simulink model "M182_Lab5"  (R2019b)
settings: Solver=VariableStepAuto  StartTime=0.0  StopTime=10000  RelTol=1e-3
libraries: simulink x1
settings Model: Creator=scjcb  LastModifiedBy=scjcb

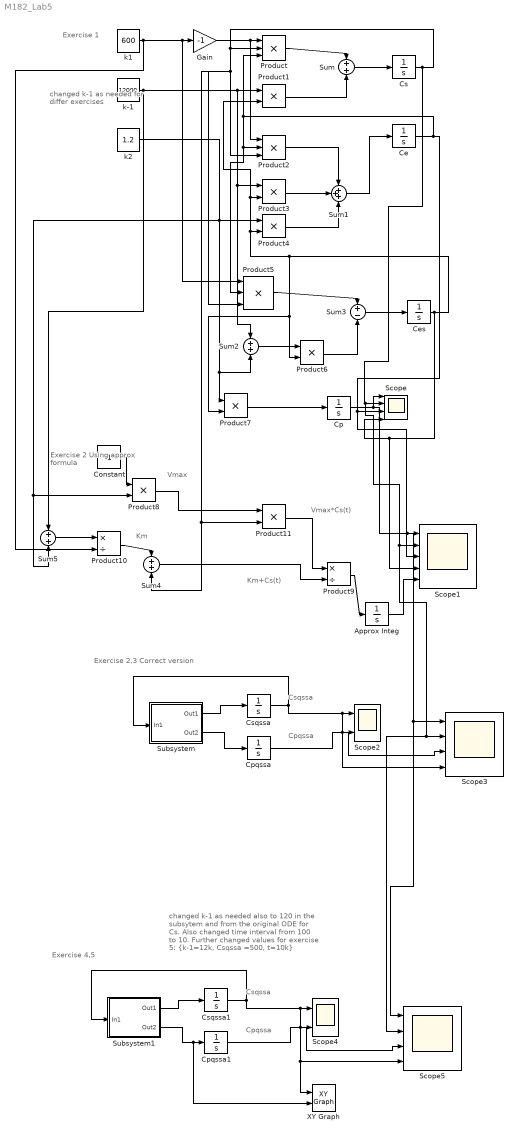
== system M182_Lab5 ==
  note: changed k-1 as needed also
      | to 120 in the subsytem and from
      | the original ODE for Cs. Also changed
      | time interval from 100 to 10.
      | Further changed values for exercise 5:
      | {k-1=12k, Csqssa =500, t=10k}
  note: changed k-1 as
      | needed for
      | differ exercises
  note: Exercise 2,3 Correct version
  note: Cpqssa
  note: Csqssa
  note: Vmax*Cs(t)
  note: Km+Cs(t)
  note: Vmax
  note: Km
  note: Exercise 2
      | Using
      | approx formula
  note: Exercise 1
  note: Cpqssa
  note: Exercise 4,5
  note: Csqssa
  Approx Integ : Integrator
  Ce : Integrator  InitialCondition=1
  Ces : Integrator
  Constant : Constant
  Cp : Integrator
  Cpqssa : Integrator
  Cpqssa1 : Integrator
  Cs : Integrator  InitialCondition=1
  Csqssa : Integrator  InitialCondition=1
  Csqssa1 : Integrator  InitialCondition=500
  Gain : Gain  Gain=-1
  Product : Product  Inputs=3
  Product1 : Product
  Product10 : Product  Inputs=*/
  Product{3..4,6..8,11} (6 alike) : Product  Inputs=**
  Product2 : Product  Inputs=***
  Product5 : Product  Inputs=***
  Product9 : Product  Inputs=*/
  Scope : Scope  NumInputPorts=4
  Scope1 : Scope  NumInputPorts=5
  Scope2 : Scope  NumInputPorts=2
  Scope3 : Scope  NumInputPorts=4
  Scope4 : Scope  NumInputPorts=2
  Scope5 : Scope  NumInputPorts=4
  Subsystem : Subsystem
  Subsystem1 : Subsystem
  Sum{,2,4..5} (4 alike) : Sum
  Sum1 : Sum  Inputs=+++
  Sum3 : Sum  Inputs=+-
  XY Graph : simulink/Sinks/XY Graph  xmin=490  xmax=510  ymin=1  ymax=1.16  st=-1
  k-1 : Constant  Value=12000
  k1 : Constant  Value=600
  k2 : Constant  Value=1.2
  wires:
  Sum/1 -> Cs/1
  Cs/1 -> Scope/2, Scope1/2, Scope5/2, Scope3/2, Product2/3, Product5/3, Product11/2, Sum4/2, Product/2
  Ce/1 -> Scope/3, Scope1/3, Product2/2, Product5/2, Product/3
  k1/1 -> Product10/2, Product5/1, Gain/1
  Gain/1 -> Product2/1, Product/1
  k-1/1 -> Sum5/1, Product3/1, Sum2/1, Product1/1
  Ces/1 -> Scope1/4, Scope/4, Product6/2, Product7/2, Product1/2, Product3/2, Product4/2
  k2/1 -> Product4/1, Product7/1, Sum2/2, Sum5/2, Product8/2
  Product2/1 -> Sum1/1
  Product3/1 -> Sum1/2
  Product4/1 -> Sum1/3
  Sum1/1 -> Ce/1
  Product1/1 -> Sum/2
  Product/1 -> Sum/1
  Sum2/1 -> Product6/1
  Product6/1 -> Sum3/2
  Product5/1 -> Sum3/1
  Sum3/1 -> Ces/1
  Product7/1 -> Cp/1
  Cp/1 -> Scope5/1, Scope3/1, Scope1/1, Scope/1
  Sum5/1 -> Product10/1
  Product10/1 -> Sum4/1
  Constant/1 -> Product8/1
  Sum4/1 -> Product9/2
  Product8/1 -> Product11/1
  Product11/1 -> Product9/1
  Product9/1 -> Approx Integ/1
  Approx Integ/1 -> Scope1/5
  Csqssa/1 -> Scope3/4, Scope2/1, Subsystem/1(In1)
  Subsystem/1(Out1) -> Csqssa/1
  Subsystem/2(Out2) -> Cpqssa/1
  Cpqssa/1 -> Scope3/3, Scope2/2
  Subsystem1/1(Out1) -> Csqssa1/1
  Csqssa1/1 -> Scope5/4, XY Graph/1, Scope4/1, Subsystem1/1(In1)
  Cpqssa1/1 -> Scope5/3, Scope4/2
  Subsystem1/2(Out2) -> XY Graph/2, Cpqssa1/1

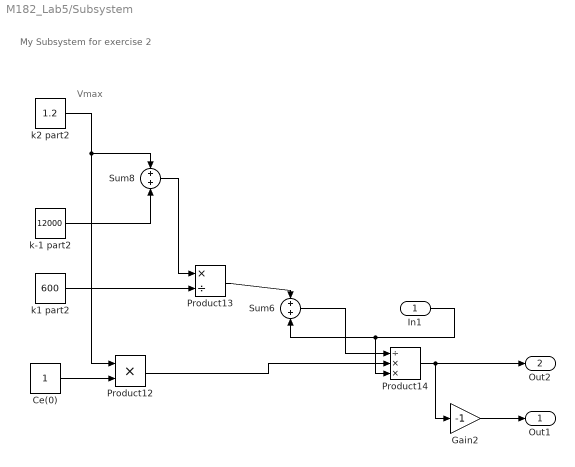
== system M182_Lab5/Subsystem ==
  note: My Subsystem for exercise 2
  note: Vmax
  In1 : Inport
  Ce(0) : Constant
  Gain2 : Gain  Gain=-1
  Product12 : Product  Inputs=**
  Product13 : Product  Inputs=*/
  Product14 : Product  Inputs=/**
  Sum6 : Sum
  Sum8 : Sum
  k-1 part2 : Constant  Value=12000
  k1 part2 : Constant  Value=600
  k2 part2 : Constant  Value=1.2
  Out1 : Outport
  Out2 : Outport  Port=2
  wires:
  k1 part2/1 -> Product13/2
  Product14/1 -> Out2/1, Gain2/1
  Sum6/1 -> Product14/1
  k-1 part2/1 -> Sum8/2
  In1/1 -> Product14/3, Sum6/2
  Gain2/1 -> Out1/1
  Ce(0)/1 -> Product12/2
  k2 part2/1 -> Sum8/1, Product12/1
  Sum8/1 -> Product13/1
  Product13/1 -> Sum6/1
  Product12/1 -> Product14/2

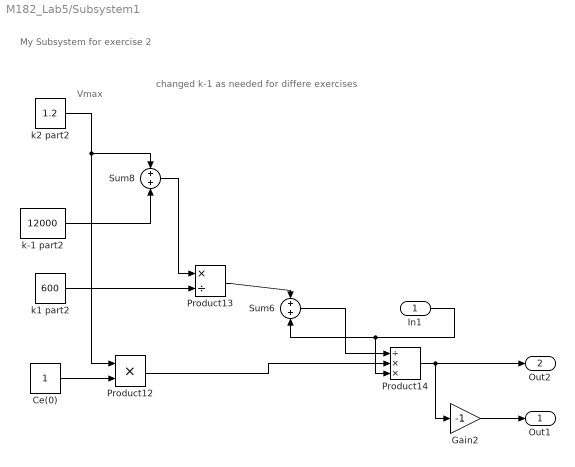
== system M182_Lab5/Subsystem1 ==
  note: changed k-1 as needed for differe exercises
  note: My Subsystem for exercise 2
  note: Vmax
  In1 : Inport
  Ce(0) : Constant
  Gain2 : Gain  Gain=-1
  Product12 : Product  Inputs=**
  Product13 : Product  Inputs=*/
  Product14 : Product  Inputs=/**
  Sum6 : Sum
  Sum8 : Sum
  k-1 part2 : Constant  Value=12000
  k1 part2 : Constant  Value=600
  k2 part2 : Constant  Value=1.2
  Out1 : Outport
  Out2 : Outport  Port=2
  wires:
  k1 part2/1 -> Product13/2
  Product14/1 -> Out2/1, Gain2/1
  Sum6/1 -> Product14/1
  k-1 part2/1 -> Sum8/2
  In1/1 -> Product14/3, Sum6/2
  Gain2/1 -> Out1/1
  Ce(0)/1 -> Product12/2
  k2 part2/1 -> Sum8/1, Product12/1
  Sum8/1 -> Product13/1
  Product13/1 -> Sum6/1
  Product12/1 -> Product14/2
